simulink subsystem "EKF_correction"  (R2021a)
settings: Solver=VariableStepAuto  StartTime=0.0  StopTime=10.0  RelTol=1e-3
undefined symbols (not defined in the file): imu1, magnitude
libraries: dspmtrx3 x3, aerolibutil x3
settings Model: Creator=Laura  LastModifiedBy=Laura

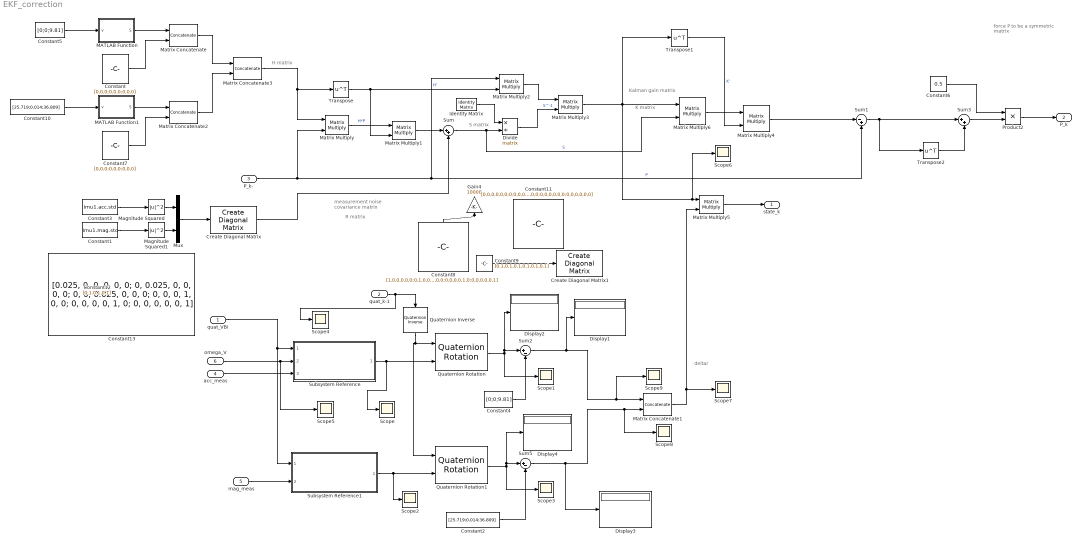
== system EKF_correction ==
  note: deltar
  note: Kalman gain matrix
  note: force P to be a symmetric matrix
  note: K matrix
  note: S matrix
  note: R matrix
  note: H matrix
  note: measurement noise covariance matrix
  quat_VBi : Inport
  quat_k-1 : Inport  Port=2
  P_k- : Inport  Port=3
  acc_meas : Inport  Port=4
  mag_meas : Inport  Port=5
  omega_V : Inport  Port=6
  Constant : Constant  Value=[0,0,0;0,0,0;0,0,0]
  Constant1 : Constant  Value=imu1.mag.std
  Constant10 : Constant  Value=[25.719;0.014;36.809]
  Constant11 : Constant  Value=[0,0,0,0,0,0;0,0,0,0,0,0;0,0,0,0,0,0;0,0,0,0,0,0;0,0,0,0,0,0;0,0,0,0,0,0]
  Constant12 : Constant  Value=[0.1,0.1,0.1]
  Constant13 : Constant  Value=[0.025, 0, 0, 0, 0, 0; 0, 0.025, 0, 0, 0, 0; 0, 0, 0.025, 0, 0, 0; 0, 0, 0, 1, 0, 0; 0, 0, 0, 0, 1, 0; 0, 0, 0, 0, 0, 1]
  Constant2 : Constant  Value=[25.719;0.014;36.809]
  Constant3 : Constant  Value=imu1.acc.std
  Constant4 : Constant  Value=[0;0;9.81]
  Constant5 : Constant  Value=[0;0;9.81]
  Constant6 : Constant  Value=0.5
  Constant7 : Constant  Value=[0,0,0;0,0,0;0,0,0]
  Constant8 : Constant  Value=[1,0,0,0,0,0;0,1,0,0,0,0;0,0,1,0,0,0;0,0,0,1,0,0;0,0,0,0,1,0;0,0,0,0,0,1]
  Constant9 : Constant  Value=[0.1,0.1,0.1,0.1,0.1,0.1]
  Create Diagonal Matrix : dspmtrx3/Create Diagonal Matrix
      settings: SourceProductBaseCode=DS
  Create Diagonal Matrix1 : dspmtrx3/Create Diagonal Matrix
      settings: SourceProductBaseCode=DS
  Display{1..4} (4 alike) : Display
  Divide : Product  Inputs=*/  Multiplication=Matrix(*)
  Gain4 : Gain  Gain=10000
  Identity Matrix : dspmtrx3/Identity Matrix  Inherit=off  N=6  Ts=1  dataType=double  isSigned=on  wordLen=16  udDataType=sfix(16)  fracBitsMode=Best precision  numFracBits=15  OutDataTypeStr=double  LastOutDataTypeStr=double
  MATLAB Function : MATLAB Function  TreatAsAtomicUnit=on
  MATLAB Function1 : MATLAB Function  TreatAsAtomicUnit=on
  Magnitude Squared : Math  Operator=magnitude^2  SaturateOnIntegerOverflow=on
  Magnitude Squared1 : Math  Operator=magnitude^2  SaturateOnIntegerOverflow=on
  Matrix Concatenate : Concatenate  Mode=Multidimensional array  ConcatenateDimension=2
  Matrix Concatenate1 : Concatenate  Mode=Multidimensional array
  Matrix Concatenate2 : Concatenate  Mode=Multidimensional array  ConcatenateDimension=2
  Matrix Concatenate3 : Concatenate  Mode=Multidimensional array
  Matrix Multiply{,1..6} (7 alike) : Product  Multiplication=Matrix(*)
  Mux : Mux  Inputs=2
  Product2 : Product
  Quaternion Inverse : aerolibutil/Quaternion Inverse
  Quaternion Rotation : aerolibutil/Quaternion Rotation
  Quaternion Rotation1 : aerolibutil/Quaternion Rotation
  Scope{,1..9} (10 alike) : Scope
  Subsystem Reference : Subsystem  ReferencedSubsystem=accSensor2CM
  Subsystem Reference1 : Subsystem  ReferencedSubsystem=magSensor2CM
  Sum : Sum  Inputs=|++
  Sum1 : Sum  Inputs=|-+
  Sum2 : Sum  Inputs=|+-
  Sum3 : Sum  Inputs=|++
  Sum5 : Sum  Inputs=|+-
  Transpose : Math  Operator=transpose  SaturateOnIntegerOverflow=on
  Transpose1 : Math  Operator=transpose  SaturateOnIntegerOverflow=on
  Transpose2 : Math  Operator=transpose  SaturateOnIntegerOverflow=on
  state_k : Outport
  P_k : Outport  Port=2
  wires:
  Constant8/1 -> Gain4/1
  Quaternion Rotation1/1 -> Scope3/1, Display4/1, Sum5/1
  mag_meas/1 -> Subsystem Reference1/2
  Matrix Multiply5/1 -> state_k/1
  Matrix Concatenate1/1 -> Scope7/1, Matrix Multiply5/2
  Sum5/1 -> Scope8/1, Matrix Concatenate1/2, Display3/1
  Sum2/1 -> Scope9/1, Matrix Concatenate1/1, Display1/1
  Constant2/1 -> Sum5/2
  Constant4/1 -> Sum2/2
  acc_meas/1 -> Subsystem Reference/3
  Matrix Multiply4/1 -> Sum1/1
  Transpose1/1 -> Matrix Multiply4/2  "K'"
  Matrix Multiply6/1 -> Matrix Multiply4/1
  Sum/1 -> Divide/2, Matrix Multiply6/2  "S"
  Magnitude Squared/1 -> Mux/1
  Magnitude Squared1/1 -> Mux/2
  Mux/1 -> Create Diagonal Matrix/1
  Sum1/1 -> Transpose2/1, Sum3/1
  Constant3/1 -> Magnitude Squared/1
  MATLAB Function/1(S) -> Matrix Concatenate/1
  Constant/1 -> Matrix Concatenate/2
  P_k-/1 -> Sum1/2, Matrix Multiply2/1, Matrix Multiply/2  "P"
  Transpose/1 -> Matrix Multiply2/2, Matrix Multiply1/2  "H'"
  Matrix Multiply1/1 -> Sum/1
  Matrix Multiply/1 -> Matrix Multiply1/1  "H*P"
  Matrix Multiply2/1 -> Matrix Multiply3/1
  Divide/1 -> Matrix Multiply3/2  "S^-1"
  Sum3/1 -> Product2/2
  Product2/1 -> P_k/1
  Constant6/1 -> Product2/1
  Transpose2/1 -> Sum3/2
  Constant5/1 -> MATLAB Function/1(v)
  Constant10/1 -> MATLAB Function1/1(v)
  MATLAB Function1/1(S) -> Matrix Concatenate2/1
  Constant7/1 -> Matrix Concatenate2/2
  Matrix Concatenate/1 -> Matrix Concatenate3/1
  Matrix Concatenate2/1 -> Matrix Concatenate3/2
  Matrix Concatenate3/1 -> Transpose/1, Matrix Multiply/1
  Identity Matrix/1 -> Divide/1
  quat_VBi/1 -> Subsystem Reference/1, Subsystem Reference1/1
  omega_V/1 -> Subsystem Reference/2, Scope5/1
  Subsystem Reference/1 -> Scope/1, Quaternion Rotation/2
  quat_k-1/1 -> Scope4/1, Quaternion Inverse/1
  Subsystem Reference1/1 -> Scope2/1, Quaternion Rotation1/2
  Quaternion Rotation/1 -> Scope1/1, Sum2/1, Display2/1
  Quaternion Inverse/1 -> Quaternion Rotation/1, Quaternion Rotation1/1
  Matrix Multiply3/1 -> Transpose1/1, Matrix Multiply6/1, Scope6/1, Matrix Multiply5/1
  Constant9/1 -> Create Diagonal Matrix1/1
  Create Diagonal Matrix/1 -> Sum/2
  Constant1/1 -> Magnitude Squared1/1

== matlab function EKF_correction/MATLAB Function1 ==
  data: v input; S output
function S = skewm(v)
% skewm forms a skew-symmetric matrix from a 3x1 vector
%
% INPUT
%              v, 3x1 vector
%
%	OUTPUT
%              S, 3x3 skew-symmetric matrix
%
%%
    x = v(1);
    y = v(2);
    z = v(3);

    S = [ 0 -z   y;
          z  0  -x;
         -y  x   0];

end

== matlab function EKF_correction/MATLAB Function ==
  data: v input; S output
function S = skewm(v)
% skewm forms a skew-symmetric matrix from a 3x1 vector
%
% INPUT
%              v, 3x1 vector
%
%	OUTPUT
%              S, 3x3 skew-symmetric matrix
%
%%
    x = v(1);
    y = v(2);
    z = v(3);

    S = [ 0 -z   y;
          z  0  -x;
         -y  x   0];

end
